simulink model "doc_qam_scatter"  (Simulink 6.0)
settings: Solver=ode45  StartTime=0.0  StopTime=250  RelTol=1e-3
undefined symbols (not defined in the file): figposition, slcm
libraries: commchan2 x1, commsink2 x1, commrandsrc2 x1, commdigbbndam2 x1
settings Model: Creator=ashivapr  LastModifiedBy=ysong  ExtModeAutoUpdateStatusClock=off
settings DataIOCC: SignalLoggingName=sigsOut
settings OptimizationCC: BlockReduction=off  BooleanDataType=off
settings DebuggingCC: CheckExecutionContextPreStartOutputMsg=on  CheckExecutionContextRuntimeOutputMsg=on  SolverPrmCheckMsg=none  InheritedTsInSrcMsg=none
settings HardwareCC: TargetUnknown=on
settings ModelReferenceCC: UpdateModelReferenceTargets=IfOutOfDate
settings GRTTargetCC: LifeSpan=inf
settings SFSimCC: SFSimApplyToAllLibs=on  SFSimBuildMode=Incremental

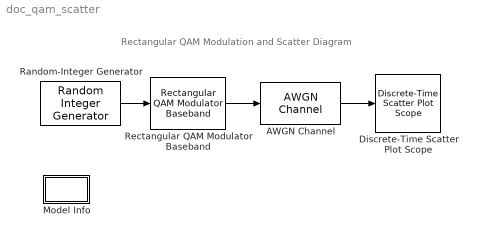
== system doc_qam_scatter ==
  note: Rectangular QAM Modulation and Scatter Diagram
  AWGN Channel : commchan2/AWGN Channel  seed=1  noiseMode="Signal to noise ratio  (Es/No)"  EbNodB=10  EsNodB=20  SNRdB=10  bitsPerSym=1  Ps=1  Tsym=.1  variance=1
  Discrete-Time Scatter Plot Scope : commsink2/Discrete-Time Scatter Plot Scope  Tag=ScatterPlot  sampPerSymb=1  offsetEye=0  numTraces=160  numNewFrames=80  LineMarkers=.  LineColors=b  fading=on  render=on  AxisGrid=on  xMin=-1.5  xMax=1.5  yMin=-1.5  yMax=1.5  inphaseLabel=In-phase Amplitude  quadratureLabel=Quadrature Amplitude  openScopeAtSimStart=on  FrameNumber=off  FigPos=figposition([2.5 55 35 35]);  figTitle=Scatter Plot  numLinesMax=8  block_type_=scatter
  Model Info : Subsystem  LoadFcn=slcm LoadBlock;  InitFcn=slcm('UpdateAllCMBlocksInThisModelInit')  EnableExecutionContextPropagation=on  mask(CMBlock){InitialSaveTempField=, InitialBlockCM=none, BlockCM=none, Frame=on, SaveTempField=, DisplayStringWithTags=Info, MaskDisplayString=Info, HorizontalTextAlignment=Center, LeftAlignmentValue=0.5, SourceBlockDiagram=doc_qam_scatter, TagMaxNumber=20, CMTag1=, CMTag2=, CMTag3=, CMTag4=, CMTag5=, CMTag6=, CMTag7=, CMTag8=, CMTag9=, CMTag10=, CMTag11=, CMTag12=, CMTag13=, CMTag14=, CMTag15=, CMTag16=, CMTag17=, CMTag18=, CMTag19=, CMTag20=}
      mask help: This block allows revision control information to be displayed within the model.
      settings: CopyFcn=slcm CopyBlock;  DeleteFcn=slcm Cancel;  PostSaveFcn=slcm('UpdateAllCMBlocksInThisModel')  NameChangeFcn=slcm Rename;  OpenFcn=commdemohelp;
      mask Display: text(str2num(LeftAlignmentValue), 0.5, MaskDisplayString, 'HorizontalAlignment', HorizontalTextAlignment)
  Random-Integer Generator : commrandsrc2/Random Integer Generator  mul=16  seed=392  Ts=.1  frameBased=off  sampPerFrame=1  orient=off
  Rectangular QAM Modulator Baseband : commdigbbndam2/Rectangular QAM Modulator Baseband  M=16  InType=Integer  Enc=Binary  PowType=Peak Power  MinDist=2  AvgPow=1  PeakPow=1  Ph=0  numSamp=1
  wires:
  AWGN Channel/1 -> Discrete-Time Scatter Plot Scope/1
  Random-Integer Generator/1 -> Rectangular QAM Modulator Baseband/1
  Rectangular QAM Modulator Baseband/1 -> AWGN Channel/1

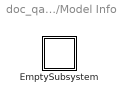
== system doc_qam_scatter/Model Info ==
  EmptySubsystem : Subsystem  EnableExecutionContextPropagation=on

== system doc_qam_scatter/Model Info/EmptySubsystem ==
